simulink model "Glider"  (R2019a)
settings: Solver=ode4  StartTime=0.0  StopTime=200.0  FixedStep=0.1  RelTol=1e-3
libraries: simulink x2
settings Model: Creator=whsteyn  LastModifiedBy=Wian
settings DataIOCC: LimitDataPoints=on  SaveFormat=Array  SignalLoggingSaveFormat=ModelDataLogs  ReturnWorkspaceOutputs=off
settings OptimizationCC: InitFltsAndDblsToZero=on  LifeSpan=inf
settings DebuggingCC: SaveWithParameterizedLinksMsg=none  UnderspecifiedInitializationDetection=Classic  MergeDetectMultiDrivingBlocksExec=none  SignalResolutionControl=TryResolveAllWithWarning  SolverPrmCheckMsg=warning  MultiTaskDSMMsg=warning  MultiTaskCondExecSysMsg=none  FcnCallInpInsideContextMsg=warning  SFUnexpectedBacktrackingDiag=warning  SFNoUnconditionalDefaultTransitionDiag=warning  SFExecutionAtInitializationDiag=none  ArithmeticOperatorsInVariantConditions=warning
settings HardwareCC: ProdBitPerPointer=32  ProdBitPerSizeT=32  ProdBitPerPtrDiffT=32  ProdLargestAtomicFloat=None  ProdIntDivRoundTo=Undefined  ProdEndianess=Unspecified  ProdWordSize=32  ProdHWDeviceType=32-bit Generic
settings ModelReferenceCC: PropagateSignalLabelsOutOfModel=off
settings SFSimCC: SimUseLocalCustomCode=off
settings RTWCC: RTWUseLocalCustomCode=off
settings CodeAppCC: StateflowObjectComments=on
settings GRTTargetCC: TargetFcnLib=ansi_tfl_tmw.mat  TargetLangStandard=C89/C90 (ANSI)  GeneratePreprocessorConditionals=Disable all  CombineOutputUpdateFcns=off  GRTInterface=on
settings ConfigComp: CovMetricSettings=dw  CovHtmlReporting=on  CovSaveCumulativeToWorkspaceVar=on  CovSaveSingleToWorkspaceVar=on  CovExternalEMLEnable=off  CovSFcnEnable=off

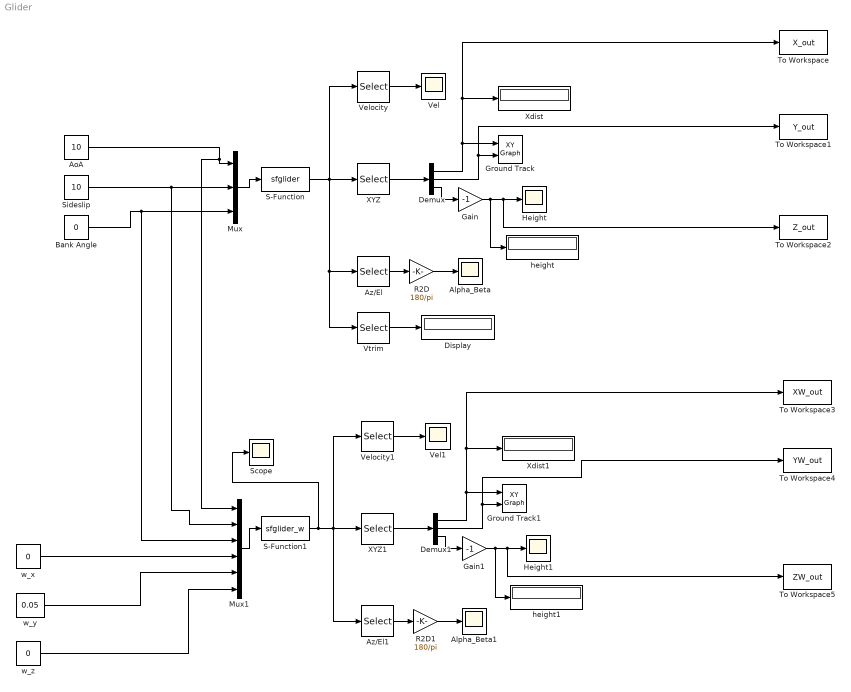
== system Glider ==
  Alpha_Beta : Scope
  Alpha_Beta1 : Scope
  AoA : Constant  Value=10
  Az/El : Selector  InputPortWidth=7  IndexOptions=Index vector (dialog)  Indices=[5,6]  OutputSizes=1
  Az/El1 : Selector  InputPortWidth=6  IndexOptions=Index vector (dialog)  Indices=[5,6]  OutputSizes=1
  Bank Angle : Constant  Value=0
  Demux : Demux  Outputs=3
  Demux1 : Demux  Outputs=3
  Display : Display
  Gain : Gain  Gain=-1
  Gain1 : Gain  Gain=-1
  Ground Track : simulink/Sinks/XY Graph  xmin=0  xmax=2500  ymin=-1000  ymax=1000  st=-1
  Ground Track1 : simulink/Sinks/XY Graph  xmin=0  xmax=2500  ymin=-1000  ymax=1000  st=-1
  Height : Scope
  Height1 : Scope
  Mux : Mux  Inputs=3
  Mux1 : Mux  Inputs=6
  R2D : Gain  Gain=180/pi
  R2D1 : Gain  Gain=180/pi
  S-Function : S-Function  FunctionName=sfglider  Parameters=10,1000.0,2.254,[0 0]  SFunctionDeploymentMode=off  EnableBusSupport=off
  S-Function1 : S-Function  FunctionName=sfglider_w  Parameters=10,1000.0,2.254,[0 0]  SFunctionDeploymentMode=off  EnableBusSupport=off
  Scope : Scope
  Sideslip : Constant  Value=10
  To Workspace : ToWorkspace  VariableName=X_out  SampleTime=-1
  To Workspace1 : ToWorkspace  VariableName=Y_out  SampleTime=-1
  To Workspace2 : ToWorkspace  VariableName=Z_out  SampleTime=-1
  To Workspace3 : ToWorkspace  VariableName=XW_out  SampleTime=-1
  To Workspace4 : ToWorkspace  VariableName=YW_out  SampleTime=-1
  To Workspace5 : ToWorkspace  VariableName=ZW_out  SampleTime=-1
  Vel : Scope
  Vel1 : Scope
  Velocity : Selector  InputPortWidth=7  IndexOptions=Index vector (dialog)  Indices=[4]  OutputSizes=1
  Velocity1 : Selector  InputPortWidth=6  IndexOptions=Index vector (dialog)  Indices=[4]  OutputSizes=1
  Vtrim : Selector  InputPortWidth=7  IndexOptions=Index vector (dialog)  Indices=[7]  OutputSizes=1
  XYZ : Selector  InputPortWidth=7  IndexOptions=Index vector (dialog)  Indices=[1:3]  OutputSizes=1
  XYZ1 : Selector  InputPortWidth=6  IndexOptions=Index vector (dialog)  Indices=[1:3]  OutputSizes=1
  Xdist : Display
  Xdist1 : Display
  height : Display
  height1 : Display
  w_x : Constant  Value=0
  w_y : Constant  Value=0.05
  w_z : Constant  Value=0
  wires:
  Mux/1 -> S-Function/1
  S-Function/1 -> Velocity/1, XYZ/1, Vtrim/1, Az/El/1
  XYZ/1 -> Demux/1
  Velocity/1 -> Vel/1
  Gain/1 -> height/1, To Workspace2/1, Height/1
  Demux/3 -> Gain/1
  Demux/1 -> To Workspace/1, Xdist/1, Ground Track/1
  Demux/2 -> To Workspace1/1, Ground Track/2
  Az/El/1 -> R2D/1
  R2D/1 -> Alpha_Beta/1
  Vtrim/1 -> Display/1
  Demux1/2 -> To Workspace4/1, Ground Track1/2
  Az/El1/1 -> R2D1/1
  Sideslip/1 -> Mux1/2, Mux/2
  AoA/1 -> Mux1/1, Mux/1
  R2D1/1 -> Alpha_Beta1/1
  Mux1/1 -> S-Function1/1
  Demux1/1 -> To Workspace3/1, Xdist1/1, Ground Track1/1
  XYZ1/1 -> Demux1/1
  Velocity1/1 -> Vel1/1
  Demux1/3 -> Gain1/1
  S-Function1/1 -> Scope/1, Velocity1/1, XYZ1/1, Az/El1/1
  Gain1/1 -> height1/1, To Workspace5/1, Height1/1
  Bank Angle/1 -> Mux1/3, Mux/3
  w_x/1 -> Mux1/4
  w_y/1 -> Mux1/5
  w_z/1 -> Mux1/6
